simulink model "TV2016"  (Simulink 8.5)
settings: Solver=FixedStepDiscrete  StartTime=0.0  StopTime=inf  FixedStep=0.001  RelTol=1e-3
PreLoadFcn:
  | FSE_Parameters
values from neighbouring files (symbols this model uses):
  car_params = Simulink_Car_params    [TV2016_parameters.m]
  i_Diff = 15.47    [TV2016_parameters.m]
  Kp = 1    [TV2016_parameters.m]
  powerLimitControl = Simulink_el    [TV2016_parameters.m]
  settings = Simulink_Settings    [TV2016_parameters.m]
  SpdC_BCC = 0    [TV2016_parameters.m]
  Speed_Neg_sat = -21    [TV2016_parameters.m]
  Speed_Pos_sat = 21    [TV2016_parameters.m]
  speedEstimation = Simulink_speedEst    [TV2016_parameters.m]
  Tn_n = 0    [TV2016_parameters.m]
  tractionControl = Simulink_tc    [TV2016_parameters.m]
  Use_Joystick = 1    [TV2016_parameters.m]
  yawRateControl = Simulink_yawRate    [TV2016_parameters.m]
libraries: CarMaker4SL x174, simulink x27, simulink_extras x14
(part 2 of 5)

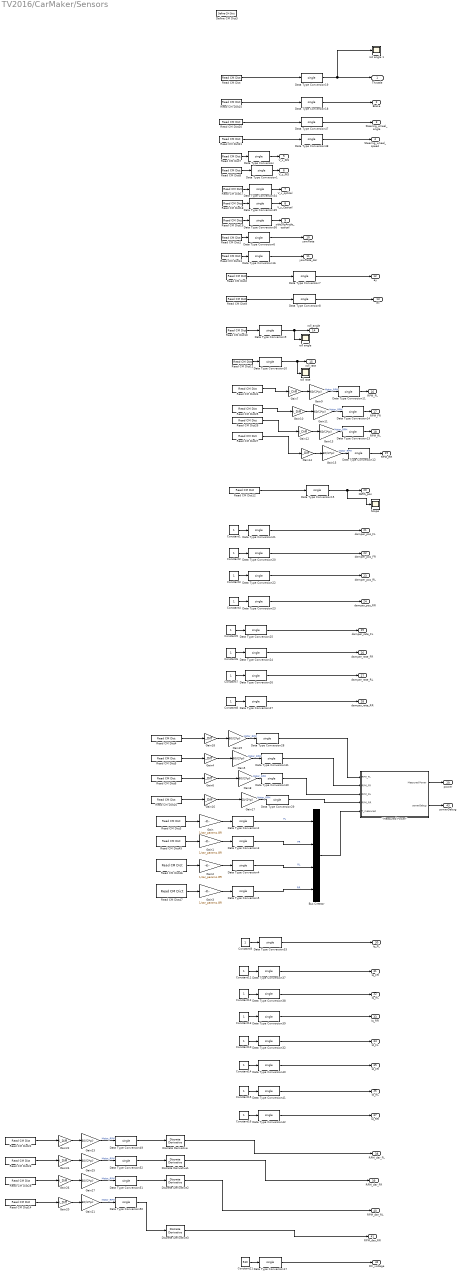
== system TV2016/CarMaker/Sensors  ==
  "\"Measured Power\"" : Subsystem
  Bus Creator : BusCreator  OutDataTypeStr=Bus: T_meas
      settings: InheritFromInputs=off
  Constant{1..16} (16 alike) : Constant
  Constant21 : Constant  Value=530
  Data Type Conversion{,1..42,47..52} (49 alike) : DataTypeConversion  OutDataTypeStr=single
  Define CM Dict3 : CarMaker4SL/Define CM Dict  xname=KERS_pos  xmono=off  xtype=Double  xdvaplace=None  xnstates=0  xfirststate=0  xinitial=0
  Discrete Derivative{,1..3} (4 alike) : simulink/Discrete/Discrete Derivative  gainval=1.0  ICPrevScaledInput=0.0  InputProcessing=Inherited  OutMin=[]  OutMax=[]  OutDataType=fixdt(1, 16)  OutScaling=2^-10  DoSatur=off
  Gain{,1..3} (4 alike) : Gain  Gain=1/car_params.GR
  Gain{4,6..7,10,12,14,16,18,20,22,24,26} (12 alike) : Gain  Gain=i_Diff
  Gain{5,8..9,11,13,15,17,19,21,23,25,27} (12 alike) : Gain  Gain=60/(2*pi)
  Read CM Dict : CarMaker4SL/Read CM Dict  xname=VC.Gas  xsync=off
  Read CM Dict1 : CarMaker4SL/Read CM Dict  xname=Vhcl.YawRate  xsync=off
  Read CM Dict10 : CarMaker4SL/Read CM Dict  xname=Vhcl.Roll  xsync=off
  Read CM Dict11 : CarMaker4SL/Read CM Dict  xname=Vhcl.RollVel  xsync=off
  Read CM Dict12 : CarMaker4SL/Read CM Dict  xname=KERS_pos  xsync=off
  Read CM Dict13 : CarMaker4SL/Read CM Dict  xname=Vhcl.YawAcc  xsync=off
  Read CM Dict14 : CarMaker4SL/Read CM Dict  xname=Car.WheelSpd_RR  xsync=off
  Read CM Dict15 : CarMaker4SL/Read CM Dict  xname=VC.Brake  xsync=off
  Read CM Dict16 : CarMaker4SL/Read CM Dict  xname=Car.WheelSpd_RR  xsync=off
  Read CM Dict17 : CarMaker4SL/Read CM Dict  xname=Car.vx  xsync=off
  Read CM Dict18 : CarMaker4SL/Read CM Dict  xname=Car.vy  xsync=off
  Read CM Dict19 : CarMaker4SL/Read CM Dict  xname=Car.SideSlipAngle  xsync=off
  Read CM Dict2 : CarMaker4SL/Read CM Dict  xname=Car.ay  xsync=off
  Read CM Dict20 : CarMaker4SL/Read CM Dict  xname=Vhcl.Steer.Ang  xsync=off
  Read CM Dict21 : CarMaker4SL/Read CM Dict  xname=Vhcl.Steer.Vel  xsync=off
  Read CM Dict22 : CarMaker4SL/Read CM Dict  xname=Car.WheelSpd_FL  xsync=off
  Read CM Dict23 : CarMaker4SL/Read CM Dict  xname=Car.WheelSpd_FR  xsync=off
  Read CM Dict24 : CarMaker4SL/Read CM Dict  xname=Car.WheelSpd_FL  xsync=off
  Read CM Dict25 : CarMaker4SL/Read CM Dict  xname=Car.WheelSpd_FR  xsync=off
  Read CM Dict26 : CarMaker4SL/Read CM Dict  xname=Car.WheelSpd_RL  xsync=off
  Read CM Dict27 : CarMaker4SL/Read CM Dict  xname=Car.WheelSpd_RR  xsync=off
  Read CM Dict28 : CarMaker4SL/Read CM Dict  xname=Car.WheelSpd_RL  xsync=off
  Read CM Dict3 : CarMaker4SL/Read CM Dict  xname=PT.WFL.Trq_Drive  xsync=off
  Read CM Dict4 : CarMaker4SL/Read CM Dict  xname=Car.WheelSpd_FL  xsync=off
  Read CM Dict45 : CarMaker4SL/Read CM Dict  xname=PT.WFR.Trq_Drive  xsync=off
  Read CM Dict46 : CarMaker4SL/Read CM Dict  xname=PT.WRL.Trq_Drive  xsync=off
  Read CM Dict47 : CarMaker4SL/Read CM Dict  xname=PT.WRR.Trq_Drive  xsync=off
  Read CM Dict5 : CarMaker4SL/Read CM Dict  xname=Car.WheelSpd_FR  xsync=off
  Read CM Dict6 : CarMaker4SL/Read CM Dict  xname=Car.WheelSpd_RL  xsync=off
  Read CM Dict7 : CarMaker4SL/Read CM Dict  xname=Car.vx  xsync=off
  Read CM Dict8 : CarMaker4SL/Read CM Dict  xname=Car.vy  xsync=off
  Read CM Dict9 : CarMaker4SL/Read CM Dict  xname=Car.ax  xsync=off
  Scope : Scope
      settings: SaveName=ScopeData77
  "roll angle " : Scope
      settings: ShowLegends=on  YMin=-17.5  YMax=17.5  SaveName=ScopeData63
  roll angle 1 : Scope
      settings: ShowLegends=on  YMin=-17.5  YMax=17.5  SaveName=ScopeData78
  roll rate : Scope
      settings: ShowLegends=on  YMin=-17.5  YMax=17.5  SaveName=ScopeData65
  "Throttle " : Outport
  "Brake " : Outport  Port=2
  "Steering_wheel_angle " : Outport  Port=3
  Steering_wheel_speed : Outport  Port=4
  V_x_INS : Outport  Port=5
  V_y_INS : Outport  Port=6
  V_x_optical : Outport  Port=7
  V_y_Optical : Outport  Port=8
  sideSlipAngle_optical : Outport  Port=9
  yawRate : Outport  Port=10
  yawRate_der : Outport  Port=11
  ay : Outport  Port=12
  "ax " : Outport  Port=13
  roll_angle : Outport  Port=14
  roll_rate : Outport  Port=15
  RPM_FL : Outport  Port=16
  RPM_FR : Outport  Port=17
  RPM_RL : Outport  Port=18
  RPM_RR : Outport  Port=19
  KERS_pos : Outport  Port=20
  damper_pos_FL : Outport  Port=21
  damper_pos_FR : Outport  Port=22
  damper_pos_RL : Outport  Port=23
  damper_pos_RR : Outport  Port=24
  damper_rate_FL : Outport  Port=25
  damper_rate_FR : Outport  Port=26
  damper_rate_RL : Outport  Port=27
  damper_rate_RR : Outport  Port=28
  power : Outport  Port=29
  Iq_FL : Outport  Port=30
  Iq_FR : Outport  Port=31
  Iq_RL : Outport  Port=32
  Iq_RR : Outport  Port=33
  Id_FL : Outport  Port=34
  Id_FR : Outport  Port=35
  Id_RL : Outport  Port=36
  Id_RR : Outport  Port=37
  RPM_der_FL : Outport  Port=38
  RPM_der_FR : Outport  Port=39
  RPM_der_RL : Outport  Port=40
  RPM_der_RR : Outport  Port=41
  DC_voltage : Outport  Port=42
  powerDebug : Outport  Port=43
  wires:
  Read CM Dict7/1 -> Data Type Conversion/1
  Read CM Dict8/1 -> Data Type Conversion1/1
  Read CM Dict1/1 -> Data Type Conversion6/1
  Data Type Conversion/1 -> V_x_INS/1
  Data Type Conversion1/1 -> V_y_INS/1
  Data Type Conversion6/1 -> yawRate/1
  Read CM Dict10/1 -> Data Type Conversion9/1
  Data Type Conversion9/1 -> "roll angle "/1, roll_angle/1
  Read CM Dict11/1 -> Data Type Conversion10/1
  Data Type Conversion10/1 -> roll rate/1, roll_rate/1
  Gain7/1 -> Gain9/1
  Read CM Dict24/1 -> Gain7/1
  Read CM Dict25/1 -> Gain10/1
  Gain10/1 -> Gain11/1
  Gain12/1 -> Gain13/1
  Gain14/1 -> Gain15/1
  Read CM Dict26/1 -> Gain12/1
  Read CM Dict27/1 -> Gain14/1
  Gain9/1 -> Data Type Conversion11/1  "Motor_RPM"
  Gain15/1 -> Data Type Conversion12/1  "Motor_RPM"
  Gain13/1 -> Data Type Conversion13/1  "Motor_RPM"
  Gain11/1 -> Data Type Conversion14/1  "Motor_RPM"
  Data Type Conversion11/1 -> RPM_FL/1
  Data Type Conversion14/1 -> RPM_FR/1
  Data Type Conversion13/1 -> RPM_RL/1
  Data Type Conversion12/1 -> RPM_RR/1
  Read CM Dict12/1 -> Data Type Conversion15/1
  Data Type Conversion15/1 -> Scope/1, KERS_pos/1
  Data Type Conversion7/1 -> ay/1
  Data Type Conversion8/1 -> "ax "/1
  Read CM Dict/1 -> Data Type Conversion19/1
  Read CM Dict15/1 -> Data Type Conversion18/1
  Data Type Conversion18/1 -> "Brake "/1
  Data Type Conversion19/1 -> roll angle 1/1, "Throttle "/1
  Data Type Conversion21/1 -> damper_pos_FL/1
  Constant1/1 -> Data Type Conversion21/1
  Data Type Conversion20/1 -> damper_pos_FR/1
  Constant2/1 -> Data Type Conversion20/1
  Data Type Conversion22/1 -> damper_pos_RL/1
  Constant3/1 -> Data Type Conversion22/1
  Data Type Conversion23/1 -> damper_pos_RR/1
  Constant4/1 -> Data Type Conversion23/1
  Data Type Conversion25/1 -> damper_rate_FL/1
  Constant5/1 -> Data Type Conversion25/1
  Data Type Conversion24/1 -> damper_rate_FR/1
  Constant6/1 -> Data Type Conversion24/1
  Data Type Conversion26/1 -> damper_rate_RL/1
  Constant7/1 -> Data Type Conversion26/1
  Data Type Conversion27/1 -> damper_rate_RR/1
  Constant8/1 -> Data Type Conversion27/1
  Read CM Dict3/1 -> Gain/1
  Read CM Dict45/1 -> Gain1/1
  Read CM Dict46/1 -> Gain2/1
  Read CM Dict47/1 -> Gain3/1
  Data Type Conversion2/1 -> Bus Creator/1  "FL"
  Data Type Conversion3/1 -> Bus Creator/2  "FR"
  Data Type Conversion4/1 -> Bus Creator/3  "RL"
  Data Type Conversion5/1 -> Bus Creator/4  "RR"
  Gain/1 -> Data Type Conversion2/1
  Gain1/1 -> Data Type Conversion3/1
  Gain2/1 -> Data Type Conversion4/1
  Gain3/1 -> Data Type Conversion5/1
  Bus Creator/1 -> "\"Measured Power\""/5(T_measured)
  Gain18/1 -> Gain19/1
  Read CM Dict4/1 -> Gain18/1
  Read CM Dict5/1 -> Gain4/1
  Gain4/1 -> Gain5/1
  Gain6/1 -> Gain8/1
  Gain16/1 -> Gain17/1
  Read CM Dict6/1 -> Gain6/1
  Read CM Dict16/1 -> Gain16/1
  Gain19/1 -> Data Type Conversion28/1  "Motor_RPM"
  Gain17/1 -> Data Type Conversion29/1  "Motor_RPM"
  Gain8/1 -> Data Type Conversion30/1  "Motor_RPM"
  Gain5/1 -> Data Type Conversion31/1  "Motor_RPM"
  Data Type Conversion29/1 -> "\"Measured Power\""/4(RPM_RR)
  Data Type Conversion30/1 -> "\"Measured Power\""/3(RPM_RL)
  Data Type Conversion31/1 -> "\"Measured Power\""/2(RPM_FR)
  Data Type Conversion28/1 -> "\"Measured Power\""/1(RPM_FL)
  "\"Measured Power\""/1("Measured Power ") -> power/1
  "\"Measured Power\""/2(powerDebug) -> powerDebug/1
  Data Type Conversion33/1 -> Iq_FL/1
  Constant9/1 -> Data Type Conversion33/1
  Data Type Conversion32/1 -> Id_FL/1
  Constant10/1 -> Data Type Conversion32/1
  Read CM Dict9/1 -> Data Type Conversion8/1
  Read CM Dict2/1 -> Data Type Conversion7/1
  Read CM Dict17/1 -> Data Type Conversion34/1
  Read CM Dict18/1 -> Data Type Conversion35/1
  Data Type Conversion34/1 -> V_x_optical/1
  Data Type Conversion35/1 -> V_y_Optical/1
  Data Type Conversion36/1 -> sideSlipAngle_optical/1
  Read CM Dict19/1 -> Data Type Conversion36/1
  Data Type Conversion37/1 -> Iq_FR/1
  Constant11/1 -> Data Type Conversion37/1
  Data Type Conversion38/1 -> Iq_RL/1
  Constant12/1 -> Data Type Conversion38/1
  Data Type Conversion39/1 -> Iq_RR/1
  Constant13/1 -> Data Type Conversion39/1
  Data Type Conversion40/1 -> Id_FR/1
  Constant14/1 -> Data Type Conversion40/1
  Data Type Conversion41/1 -> Id_RL/1
  Constant15/1 -> Data Type Conversion41/1
  Data Type Conversion42/1 -> Id_RR/1
  Constant16/1 -> Data Type Conversion42/1
  Read CM Dict20/1 -> Data Type Conversion47/1
  Read CM Dict21/1 -> Data Type Conversion48/1
  Data Type Conversion47/1 -> "Steering_wheel_angle "/1
  Data Type Conversion48/1 -> Steering_wheel_speed/1
  Data Type Conversion16/1 -> yawRate_der/1
  Read CM Dict13/1 -> Data Type Conversion16/1
  Data Type Conversion17/1 -> DC_voltage/1
  Constant21/1 -> Data Type Conversion17/1
  Gain22/1 -> Gain23/1
  Read CM Dict22/1 -> Gain22/1
  Read CM Dict23/1 -> Gain24/1
  Gain24/1 -> Gain25/1
  Gain26/1 -> Gain27/1
  Gain20/1 -> Gain21/1
  Read CM Dict28/1 -> Gain26/1
  Read CM Dict14/1 -> Gain20/1
  Gain23/1 -> Data Type Conversion49/1  "Motor_RPM"
  Gain21/1 -> Data Type Conversion50/1  "Motor_RPM"
  Gain27/1 -> Data Type Conversion51/1  "Motor_RPM"
  Gain25/1 -> Data Type Conversion52/1  "Motor_RPM"
  Data Type Conversion50/1 -> Discrete Derivative3/1
  Data Type Conversion51/1 -> Discrete Derivative2/1
  Data Type Conversion52/1 -> Discrete Derivative1/1
  Data Type Conversion49/1 -> Discrete Derivative/1
  Discrete Derivative/1 -> RPM_der_FL/1
  Discrete Derivative1/1 -> RPM_der_FR/1
  Discrete Derivative2/1 -> RPM_der_RL/1
  Discrete Derivative3/1 -> RPM_der_RR/1

== system TV2016/CarMaker/VehicleControl ==
  note: <Your model here>
  note: When implementing a vehicle control model,
      | be sure to add '-disablevehiclecontrol' to the command line arguments
      | in the CarMaker Model Configuration block.
      | Otherwise your model will possibly not see the original DrivMan signals
      | on its inputs, but those of a currently activated C-coded vehicle control model instead.
  Sync_In : Inport
  DrivMan.In : Inport  Port=2
  Bus Creator2 : BusCreator  Inputs=2
  CreateBus Vhcl.Misc : Subsystem
  CreateBus Vhcl.Wheel.In : Subsystem
  CreateBus VhclCtrl : Subsystem
  CreateBus VhclCtrl.PT : Subsystem
  CreateBus VhclCtrl.Steering : Subsystem
  Demux2 : Demux  Outputs=2
  VehicleControl : S-Function  FunctionName=CM_Sfun  Parameters='VehicleControl'
  VehicleControlUpd : S-Function  FunctionName=CM_Sfun  Parameters='VehicleControlUpd'
  Sync_Out : Outport
  Vhcl.Model.Source : Outport  Port=2
  VhclCtrl.Steering : Outport  Port=3
  Vhcl.Wheel.In : Outport  Port=4
  Vhcl.Misc : Outport  Port=5
  VhclCtrl.Brake : Outport  Port=6
  VhclCtrl.PT : Outport  Port=7
  wires:
  CreateBus VhclCtrl/1(Out) -> VehicleControlUpd/2
  VehicleControl/2 -> CreateBus VhclCtrl/1(In)
  VehicleControlUpd/2 -> Vhcl.Model.Source/1
  VehicleControlUpd/4 -> CreateBus Vhcl.Wheel.In/1(In1)
  VehicleControlUpd/5 -> CreateBus Vhcl.Misc/1(In1)
  VehicleControlUpd/6 -> Demux2/1
  VehicleControlUpd/7 -> CreateBus VhclCtrl.PT/1(In1)
  VehicleControlUpd/3 -> CreateBus VhclCtrl.Steering/1(In1)
  CreateBus Vhcl.Misc/1(Out1) -> Vhcl.Misc/1
  CreateBus Vhcl.Wheel.In/1(Out1) -> Vhcl.Wheel.In/1
  DrivMan.In/1 -> VehicleControl/2
  VehicleControl/1 -> VehicleControlUpd/1
  Sync_In/1 -> VehicleControl/1
  CreateBus VhclCtrl.PT/1(Out1) -> VhclCtrl.PT/1
  Bus Creator2/1 -> VhclCtrl.Brake/1
  CreateBus VhclCtrl.Steering/1(Out1) -> VhclCtrl.Steering/1
  VehicleControlUpd/1 -> Sync_Out/1
  Demux2/2 -> Bus Creator2/2  "VhclCtrl BrakePark"
  Demux2/1 -> Bus Creator2/1  "VhclCtrl Brake"

== system TV2016/CarMaker/Control_System /Control  ==
  "States " : Inport
  Bus Creator : BusCreator  OutDataTypeStr=Bus: Ti_lim  NonVirtualBus=on
      settings: InheritFromInputs=off
  Bus Selector : BusSelector  OutputSignals=FL,FR,RL,RR
  "Power Limit Torque Reduction Controller " : Subsystem
  Product{1..3,5} (4 alike) : Product
  Red factor : Scope
      settings: ShowLegends=on  TimeRange=10  YMin=0.625  YMax=1  SaveName=ScopeData26
  Red factor1 : Scope
      settings: ShowLegends=on  TimeRange=10  YMin=21  YMax=21  SaveName=ScopeData45
  Red factor2 : Scope
      settings: ShowLegends=on  TimeRange=10  YMin=19.95  YMax=22.05  SaveName=ScopeData58
  "Slip Rate Control " : Subsystem
  Throttle / Brake Mapping : Subsystem
  "Torque allocation " : Subsystem
  "Yaw Rate Controller " : Subsystem
  Ti_lim : Outport
  Mz_ref : Outport  Port=2
  T_req : Outport  Port=3
  r_ref : Outport  Port=4
  Mz_error : Outport  Port=5
  wires:
  "Yaw Rate Controller "/4(Mz_ref) -> Mz_ref/1, "Torque allocation "/1(Mz_ref)
  "States "/1 -> "Yaw Rate Controller "/1(States), "Slip Rate Control "/2("States "), "Power Limit Torque Reduction Controller "/1(states), "Torque allocation "/3("States "), Throttle / Brake Mapping/1("states ")
  "Torque allocation "/1(Ti_lim) -> "Slip Rate Control "/1(Ti_ref)
  Throttle / Brake Mapping/1(T_req) -> "Slip Rate Control "/3(T_req), "Torque allocation "/2(T_req), T_req/1
  "Yaw Rate Controller "/1("r_ref ") -> r_ref/1  "r_ref"
  "Slip Rate Control "/1(Ti_lim) -> Bus Selector/1
  Bus Selector/4 -> Product3/2, Red factor1/1  "<RR>"
  Bus Selector/3 -> Product1/2  "<RL>"
  Bus Selector/2 -> Product2/2  "<FR>"
  Bus Selector/1 -> Product5/2  "<FL>"
  Product5/1 -> Bus Creator/1  "FL"
  Product2/1 -> Bus Creator/2  "FR"
  Product1/1 -> Bus Creator/3  "RL"
  Product3/1 -> Red factor2/1, Bus Creator/4  "RR"
  "Power Limit Torque Reduction Controller "/1(Reduction Factor) -> Product2/1, Product5/1, Product1/1, Product3/1, Red factor/1
  Bus Creator/1 -> Ti_lim/1
  "Torque allocation "/2("Mz_error ") -> "Yaw Rate Controller "/2("Mz_error "), Mz_error/1

== system TV2016/CarMaker/Control_System /Output Interface  ==
  states : Inport
  Ti_lim : Inport  Port=2
  MATLAB Function : MATLAB Function  TreatAsAtomicUnit=on
  "Ti_pos " : Outport
  Ti_neg : Outport  Port=2
  wi_setpoints : Outport  Port=3
  wires:
  MATLAB Function/2(Ti_neg) -> Ti_neg/1
  Ti_lim/1 -> MATLAB Function/1(Ti)
  MATLAB Function/1(Ti_pos) -> "Ti_pos "/1
  MATLAB Function/3(wi_setpoints) -> wi_setpoints/1
  states/1 -> MATLAB Function/2(states)

== system TV2016/CarMaker/Debug Information /Motor Rpm log   ==
  Abs : Abs
  Discrete Derivative : simulink/Discrete/Discrete Derivative  gainval=1.0  ICPrevScaledInput=0.0  InputProcessing=Inherited  OutMin=[]  OutMax=[]  OutDataType=fixdt(1, 16)  OutScaling=2^-10  DoSatur=off
  Fl_derivate : Scope
      settings: ShowLegends=on  TimeRange=3.722  YMin=0  YMax=10000  SaveName=ScopeData57
  Gain{7,10,12,14} (4 alike) : Gain  Gain=i_Diff
  Gain{9,11,13,15} (4 alike) : Gain  Gain=60/(2*pi)
  Mux1 : Mux
  Rate Transition : RateTransition  OutPortSampleTime=settings.control_system_sample_time
  Read CM Dict24 : CarMaker4SL/Read CM Dict  xname=Car.WheelSpd_FL  xsync=off
  Read CM Dict25 : CarMaker4SL/Read CM Dict  xname=Car.WheelSpd_FR  xsync=off
  Read CM Dict26 : CarMaker4SL/Read CM Dict  xname=Car.WheelSpd_RL  xsync=off
  Read CM Dict27 : CarMaker4SL/Read CM Dict  xname=Car.WheelSpd_RR  xsync=off
  Saturation : Saturate  UpperLimit=50000
  To File : ToFile  Filename=MAT_files\MotorRPMS.mat  MatrixName=MotorRpms  SaveFormat=Timeseries
  eng rot : Scope
      settings: ShowLegends=on  TimeRange=0.03226232678936204  YMin=358.5090361445784  YMax=366.6415662650603  SaveName=ScopeData55
  wires:
  Gain7/1 -> Gain9/1
  Gain9/1 -> Mux1/1, Rate Transition/1  "Motor_RPM"
  Read CM Dict24/1 -> Gain7/1
  Read CM Dict25/1 -> Gain10/1
  Gain10/1 -> Gain11/1
  Gain11/1 -> Mux1/2  "Motor_RPM"
  Gain12/1 -> Gain13/1
  Gain13/1 -> Mux1/3  "Motor_RPM"
  Gain14/1 -> Gain15/1
  Gain15/1 -> Mux1/4  "Motor_RPM"
  Read CM Dict26/1 -> Gain12/1
  Read CM Dict27/1 -> Gain14/1
  Mux1/1 -> eng rot/1, To File/1
  Discrete Derivative/1 -> Abs/1
  Abs/1 -> Saturation/1
  Saturation/1 -> Fl_derivate/1
  Rate Transition/1 -> Discrete Derivative/1

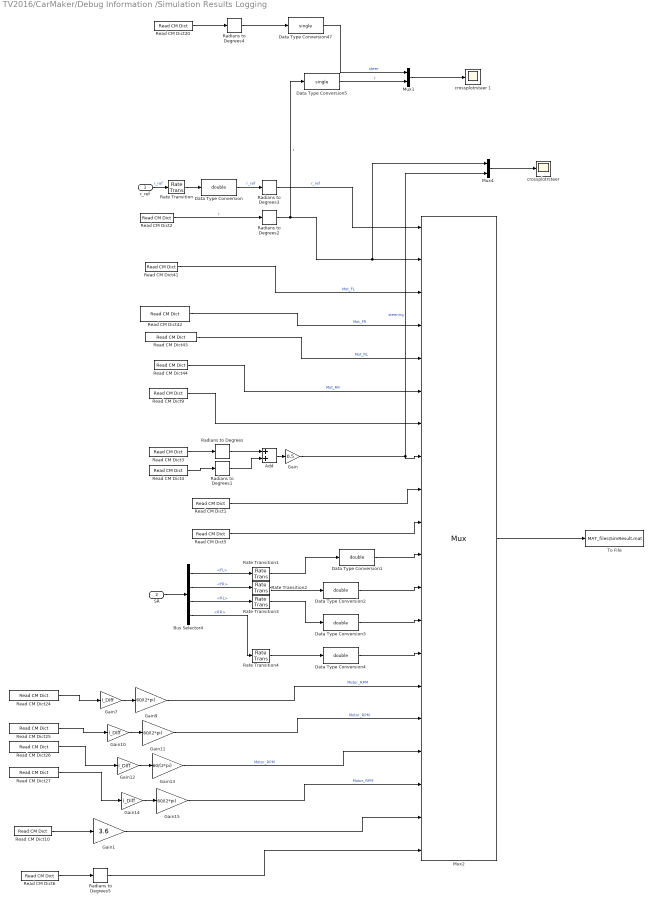
== system TV2016/CarMaker/Debug Information /Simulation Results Logging ==
  r_ref : Inport
  SR : Inport  Port=2
  Add : Sum
  Bus Selector4 : BusSelector  OutputSignals=FL,FR,RL,RR
  Data Type Conversion{,1..4} (5 alike) : DataTypeConversion  OutDataTypeStr=double
  Data Type Conversion47 : DataTypeConversion  OutDataTypeStr=single
  Data Type Conversion5 : DataTypeConversion  OutDataTypeStr=single
  Gain : Gain  Gain=0.5
  Gain1 : Gain  Gain=3.6
  Gain{7,10,12,14} (4 alike) : Gain  Gain=i_Diff
  Gain{9,11,13,15} (4 alike) : Gain  Gain=60/(2*pi)
  Mux1 : Mux  Inputs=2
  Mux2 : Mux  Inputs=20
  Mux4 : Mux  Inputs=2
  Radians to Degrees{,1..5} (6 alike) : simulink_extras/Transformations/Radians to Degrees
  Rate Transition{,1..4} (5 alike) : RateTransition  OutPortSampleTime=0.001
  Read CM Dict1 : CarMaker4SL/Read CM Dict  xname=Vhcl.Fr1.x  xsync=off
  Read CM Dict10 : CarMaker4SL/Read CM Dict  xname=Car.vx  xsync=off
  Read CM Dict2 : CarMaker4SL/Read CM Dict  xname=Car.YawRate  xsync=off
  Read CM Dict20 : CarMaker4SL/Read CM Dict  xname=Vhcl.Steer.Ang  xsync=off
  Read CM Dict24 : CarMaker4SL/Read CM Dict  xname=Car.WheelSpd_FL  xsync=off
  Read CM Dict25 : CarMaker4SL/Read CM Dict  xname=Car.WheelSpd_FR  xsync=off
  Read CM Dict26 : CarMaker4SL/Read CM Dict  xname=Car.WheelSpd_RL  xsync=off
  Read CM Dict27 : CarMaker4SL/Read CM Dict  xname=Car.WheelSpd_RR  xsync=off
  Read CM Dict3 : CarMaker4SL/Read CM Dict  xname=Car.CFR.rz  xsync=off
  Read CM Dict4 : CarMaker4SL/Read CM Dict  xname=Car.CFL.rz  xsync=off
  Read CM Dict41 : CarMaker4SL/Read CM Dict  xname=PT.WFL.Trq_Drive  xsync=off
  Read CM Dict42 : CarMaker4SL/Read CM Dict  xname=PT.WFR.Trq_Drive  xsync=off
  Read CM Dict43 : CarMaker4SL/Read CM Dict  xname=PT.WRL.Trq_Drive  xsync=off
  Read CM Dict44 : CarMaker4SL/Read CM Dict  xname=PT.WRR.Trq_Drive  xsync=off
  Read CM Dict5 : CarMaker4SL/Read CM Dict  xname=Vhcl.Fr1.y  xsync=off
  Read CM Dict6 : CarMaker4SL/Read CM Dict  xname=Vhcl.Steer.Ang  xsync=off
  Read CM Dict9 : CarMaker4SL/Read CM Dict  xname=Car.ay  xsync=off
  To File : ToFile  Filename=MAT_files\SimResult.mat  MatrixName=sim  SaveFormat=Timeseries
  "crossplotrsteer " : Scope
      settings: ShowLegends=on  TimeRange=0.01155166537365709  YMin=3.631313131313132  YMax=5.196969696969697  SaveName=ScopeData76
  crossplotrsteer 1 : Scope
      settings: ShowLegends=on  TimeRange=0.6169191083805927  YMin=-0.9397630019749759  YMax=0.9205440761112005  SaveName=ScopeData32
  wires:
  r_ref/1 -> Rate Transition/1  "r_ref"
  Read CM Dict2/1 -> Radians to Degrees2/1  "r"
  Data Type Conversion/1 -> Radians to Degrees3/1  "r_ref"
  Read CM Dict42/1 -> Mux2/4  "Mot_FR"
  Read CM Dict43/1 -> Mux2/5  "Mot_RL"
  Read CM Dict41/1 -> Mux2/3  "Mot_FL"
  Read CM Dict44/1 -> Mux2/6  "Mot_RR"
  Read CM Dict9/1 -> Mux2/7
  Read CM Dict3/1 -> Radians to Degrees/1
  Read CM Dict4/1 -> Radians to Degrees1/1
  Radians to Degrees/1 -> Add/1
  Radians to Degrees1/1 -> Add/2
  Radians to Degrees2/1 -> Mux4/1, Mux2/2, Data Type Conversion5/1  "r"
  Radians to Degrees3/1 -> Mux2/1  "r_ref"
  Add/1 -> Gain/1
  Mux2/1 -> To File/1
  Read CM Dict1/1 -> Mux2/9
  Read CM Dict5/1 -> Mux2/10
  Rate Transition/1 -> Data Type Conversion/1
  Mux4/1 -> "crossplotrsteer "/1
  Gain/1 -> Mux2/8, Mux4/2  "steering"
  Bus Selector4/1 -> Rate Transition1/1  "<FL>"
  Bus Selector4/2 -> Rate Transition2/1  "<FR>"
  Bus Selector4/3 -> Rate Transition3/1  "<RL>"
  Bus Selector4/4 -> Rate Transition4/1  "<RR>"
  SR/1 -> Bus Selector4/1
  Rate Transition1/1 -> Data Type Conversion1/1
  Rate Transition2/1 -> Data Type Conversion2/1
  Rate Transition3/1 -> Data Type Conversion3/1
  Rate Transition4/1 -> Data Type Conversion4/1
  Data Type Conversion1/1 -> Mux2/11
  Data Type Conversion2/1 -> Mux2/12
  Data Type Conversion3/1 -> Mux2/13
  Data Type Conversion4/1 -> Mux2/14
  Gain7/1 -> Gain9/1
  Gain9/1 -> Mux2/15  "Motor_RPM"
  Read CM Dict24/1 -> Gain7/1
  Read CM Dict25/1 -> Gain10/1
  Gain10/1 -> Gain11/1
  Gain11/1 -> Mux2/16  "Motor_RPM"
  Gain12/1 -> Gain13/1
  Gain13/1 -> Mux2/17  "Motor_RPM"
  Gain14/1 -> Gain15/1
  Gain15/1 -> Mux2/18  "Motor_RPM"
  Read CM Dict26/1 -> Gain12/1
  Read CM Dict27/1 -> Gain14/1
  Read CM Dict10/1 -> Gain1/1
  Gain1/1 -> Mux2/19
  Read CM Dict20/1 -> Radians to Degrees4/1
  Data Type Conversion47/1 -> Mux1/1  "steer"
  Mux1/1 -> crossplotrsteer 1/1
  Radians to Degrees4/1 -> Data Type Conversion47/1
  Data Type Conversion5/1 -> Mux1/2  "r"
  Read CM Dict6/1 -> Radians to Degrees5/1
  Radians to Degrees5/1 -> Mux2/20

== system TV2016/CarMaker/Estimations/EstimateVx ==
  sensors : Inport
  Fz_est : Inport  Port=2
  velocity_Estimation : MATLAB Function  TreatAsAtomicUnit=on
  v_x_est : Outport
  wires:
  sensors/1 -> velocity_Estimation/1(sensors)
  Fz_est/1 -> velocity_Estimation/2(normalForces)
  velocity_Estimation/1(V_est_x) -> v_x_est/1

== system TV2016/CarMaker/Estimations/Fx_Estimation ==
  sensors : Inport
  T_CM : Inport  Port=2
  EstimateFx : MATLAB Function  TreatAsAtomicUnit=on
  Fx : Outport
  wires:
  sensors/1 -> EstimateFx/1(sensors)
  EstimateFx/1(Fx) -> Fx/1
  T_CM/1 -> EstimateFx/2(T_CM)

== system TV2016/CarMaker/Estimations/Fz_Estimation ==
  sensors : Inport
  v_x : Inport  Port=2
  Bus Selector : BusSelector  OutputSignals=damper_rate_FL,damper_rate_FR,damper_rate_RL,damper_rate_RR
  Constant : Constant  Value=settings.select_Fz_est_method
  DamperRateLookup{,1..3} (4 alike) : Lookup_n-D  NumberOfTableDimensions=1  BreakpointsForDimension1=single([-250,0,250]);  Table=single([-900,0,900]);  InternalRulePriority=Speed  RndMeth=Simplest  InputSameDT=on
  FzEstDamper : MATLAB Function  TreatAsAtomicUnit=on
  FzEstLoadTransfer : MATLAB Function  TreatAsAtomicUnit=on
  Index Vector : MultiPortSwitch  Inputs=2
  Fz_est : Outport
  Fz_LoadTransfer_est : Outport  Port=2
  Fz_damper_est : Outport  Port=3
  wires:
  sensors/1 -> FzEstDamper/1(sensors), Bus Selector/1, FzEstLoadTransfer/1(sensor)
  FzEstLoadTransfer/1(Fz_loadTransfer_est) -> Fz_LoadTransfer_est/1, Index Vector/2
  DamperRateLookup/1 -> FzEstDamper/2(Fz_damp_FL)  "Fz_damp_FL"
  Bus Selector/1 -> DamperRateLookup/1  "<damper_rate_FL>"
  Bus Selector/2 -> DamperRateLookup1/1  "<damper_rate_FR>"
  Bus Selector/3 -> DamperRateLookup2/1  "<damper_rate_RL>"
  Bus Selector/4 -> DamperRateLookup3/1  "<damper_rate_RR>"
  DamperRateLookup1/1 -> FzEstDamper/3(Fz_damp_FR)
  DamperRateLookup2/1 -> FzEstDamper/4(Fz_damp_RL)
  DamperRateLookup3/1 -> FzEstDamper/5(Fz_damp_RR)
  FzEstDamper/1(Fz_damper_est) -> Index Vector/3, Fz_damper_est/1
  Constant/1 -> Index Vector/1
  Index Vector/1 -> Fz_est/1
  v_x/1 -> FzEstLoadTransfer/2(vx)

== system TV2016/CarMaker/Estimations/RPM_to_linearVelocity ==
  sensors : Inport
  meanWheelAngle : Inport  Port=2
  whl_v_calculation : MATLAB Function  TreatAsAtomicUnit=on
  whl_speed : Outport
  wires:
  whl_v_calculation/1(whl_speed) -> whl_speed/1
  sensors/1 -> whl_v_calculation/1(sensors)
  meanWheelAngle/1 -> whl_v_calculation/2(meanWheelAngle)

== system TV2016/CarMaker/Estimations/SR_Calculation ==
  v_x : Inport
  whl_v : Inport  Port=2
  sensorInput : Inport  Port=3
  Slip ratio : MATLAB Function  TreatAsAtomicUnit=on
  SR : Outport
  wires:
  v_x/1 -> Slip ratio/1(V_x)
  Slip ratio/1(SR) -> SR/1
  whl_v/1 -> Slip ratio/2(whl_v)
  sensorInput/1 -> Slip ratio/3(sensor)

== system TV2016/CarMaker/Estimations/calculateMeanWheelAngle ==
  sensorInput : Inport
  calculateWheelangleandSpeed : MATLAB Function  TreatAsAtomicUnit=on
  mean_wheel_angle : Outport
  mean_wheel_speed : Outport  Port=2
  wires:
  sensorInput/1 -> calculateWheelangleandSpeed/1(sensor)
  calculateWheelangleandSpeed/1(mean_wheel_angle) -> mean_wheel_angle/1
  calculateWheelangleandSpeed/2(mean_wheel_speed) -> mean_wheel_speed/1

== system TV2016/CarMaker/Estimations/createStateBus ==
  mean_wheel_angle : Inport
  mean_wheel_speed : Inport  Port=2
  Fz_CM : Inport  Port=3
  Fx : Inport  Port=4
  sensors : Inport  Port=5
  Fz_est : Inport  Port=6
  whl_speed_cog : Inport  Port=7
  v_x : Inport  Port=8
  v_y : Inport  Port=9
  SR : Inport  Port=10
  frictionCoefficient : Inport  Port=11
  Bus Creator1 : BusCreator  Inputs=35  OutDataTypeStr=Bus: States  NonVirtualBus=on
      settings: InheritFromInputs=off
  Bus Selector{,2..4} (4 alike) : BusSelector  OutputSignals=FL,FR,RL,RR
  Bus Selector1 : BusSelector  OutputSignals=Input_throttle,Input_brake,KERS_pos,sideSlipAngle_optical,yawRate,yawRate_der,ax,ay,RPM_FL,RPM_FR,RPM_RL,RPM_RR,power,DC_voltage
  Constant : Constant  Value=settings.use_estimated_Fz
  Index Vector : MultiPortSwitch  DataPortOrder=Zero-based contiguous  Inputs=2  zeroidx=on
  states : Outport
  wires:
  sensors/1 -> Bus Selector1/1
  Fz_est/1 -> Index Vector/3
  Fz_CM/1 -> Index Vector/2
  Constant/1 -> Index Vector/1
  Index Vector/1 -> Bus Selector/1
  whl_speed_cog/1 -> Bus Selector2/1
  Fx/1 -> Bus Selector3/1
  SR/1 -> Bus Selector4/1
  Bus Creator1/1 -> states/1
  Bus Selector1/10 -> Bus Creator1/10  "<RPM_FR>"
  Bus Selector1/9 -> Bus Creator1/9  "<RPM_FL>"
  Bus Selector1/11 -> Bus Creator1/11  "<RPM_RL>"
  Bus Selector1/8 -> Bus Creator1/8  "<ay>"
  Bus Selector1/12 -> Bus Creator1/12  "<RPM_RR>"
  Bus Selector1/7 -> Bus Creator1/7  "<ax>"
  Bus Selector1/13 -> Bus Creator1/13  "<power>"
  Bus Selector1/6 -> Bus Creator1/6  "<yawRate_der>"
  Bus Selector1/14 -> Bus Creator1/14  "<DC_voltage>"
  Bus Selector1/5 -> Bus Creator1/5  "<yawRate>"
  Bus Selector1/4 -> Bus Creator1/4  "<sideSlipAngle_optical>"
  Bus Selector1/3 -> Bus Creator1/3  "<KERS_pos>"
  Bus Selector1/2 -> Bus Creator1/2  "<Input_brake>"
  Bus Selector1/1 -> Bus Creator1/1  "<Input_throttle>"
  mean_wheel_angle/1 -> Bus Creator1/15
  mean_wheel_speed/1 -> Bus Creator1/16
  v_x/1 -> Bus Creator1/17
  v_y/1 -> Bus Creator1/18
  Bus Selector/1 -> Bus Creator1/23  "<FL>"
  Bus Selector/2 -> Bus Creator1/24  "<FR>"
  Bus Selector/3 -> Bus Creator1/25  "<RL>"
  Bus Selector/4 -> Bus Creator1/26  "<RR>"
  Bus Selector2/1 -> Bus Creator1/27  "<FL>"
  Bus Selector2/2 -> Bus Creator1/28  "<FR>"
  Bus Selector2/3 -> Bus Creator1/29  "<RL>"
  Bus Selector2/4 -> Bus Creator1/30  "<RR>"
  Bus Selector4/1 -> Bus Creator1/31  "<FL>"
  Bus Selector4/2 -> Bus Creator1/32  "<FR>"
  Bus Selector4/3 -> Bus Creator1/33  "<RL>"
  Bus Selector4/4 -> Bus Creator1/34  "<RR>"
  Bus Selector3/1 -> Bus Creator1/19  "<FL>"
  Bus Selector3/2 -> Bus Creator1/20  "<FR>"
  Bus Selector3/3 -> Bus Creator1/21  "<RL>"
  Bus Selector3/4 -> Bus Creator1/22  "<RR>"
  frictionCoefficient/1 -> Bus Creator1/35

== system TV2016/CarMaker/Estimations/friction_estimation ==
  Fx : Inport
  SR : Inport  Port=2
  Fz : Inport  Port=3
  estimateFrictionCoefficient : MATLAB Function  TreatAsAtomicUnit=on
  mu : Outport
  normLongTireForce : Outport  Port=2
  wires:
  Fx/1 -> estimateFrictionCoefficient/1(Fx)
  Fz/1 -> estimateFrictionCoefficient/2(Fz)
  SR/1 -> estimateFrictionCoefficient/3(SR)
  estimateFrictionCoefficient/1(mu) -> mu/1
  estimateFrictionCoefficient/2(normLongTireForce) -> normLongTireForce/1

== system TV2016/CarMaker/Estimations/selectVelocity ==
  v_est_x : Inport
  sensors : Inport  Port=2
  Bus Selector : BusSelector  OutputSignals=V_x_INS,V_x_optical
  Bus Selector1 : BusSelector  OutputSignals=V_y_INS,V_y_optical
  Constant1 : Constant  Value=settings.select_velocity_vx
  Constant2 : Constant  Value=settings.select_velocity_vy
  Index Vector : MultiPortSwitch
  Index Vector1 : MultiPortSwitch  DataPortOrder=Specify indices  Inputs=2  DataPortIndices={2,3}
  v_x : Outport
  v_y : Outport  Port=2
  wires:
  Constant1/1 -> Index Vector/1
  v_est_x/1 -> Index Vector/2
  sensors/1 -> Bus Selector1/1, Bus Selector/1
  Bus Selector/1 -> Index Vector/3  "<V_x_INS>"
  Bus Selector/2 -> Index Vector/4  "<V_x_optical>"
  Index Vector/1 -> v_x/1
  Constant2/1 -> Index Vector1/1
  Bus Selector1/1 -> Index Vector1/2  "<V_y_INS>"
  Bus Selector1/2 -> Index Vector1/3  "<V_y_optical>"
  Index Vector1/1 -> v_y/1

== system TV2016/CarMaker/IPG Vehicle/Brake ==
  note: <Your model here>
  note: When replacing the entire braking system,
      | be sure to add '-disablebrake' to the command line arguments
      | in the CarMaker Model Configuration block.
  Sync_In : Inport
  Brake.IF.In : Inport  Port=2
  VhclCtrl.Brake : Inport  Port=3
  Brake : S-Function  FunctionName=CM_Sfun  Parameters='Brake'
  BrakeUpd : S-Function  FunctionName=CM_Sfun  Parameters='BrakeUpd'
  BusCreator : BusCreator  Inputs=12
  CreateBus Vhcl.Wheel.PT : Subsystem
  Demux : Demux  Outputs=12
  Sync_Out : Outport
  Vhcl.Wheel.PT : Outport  Port=2
  wires:
  BrakeUpd/1 -> Sync_Out/1
  Brake/1 -> BrakeUpd/1  "Sync"
  Brake.IF.In/1 -> Brake/2
  VhclCtrl.Brake/1 -> Brake/3
  Brake/2 -> Demux/1
  BusCreator/1 -> BrakeUpd/2
  Sync_In/1 -> Brake/1
  Demux/12 -> BusCreator/12  "Brake IF Trq_Reg_trg RR"
  Demux/11 -> BusCreator/11  "Brake IF Trq_Reg_trg RL"
  Demux/10 -> BusCreator/10  "Brake IF Trq_Reg_trg FR"
  Demux/9 -> BusCreator/9  "Brake IF Trq_Reg_trg FL"
  Demux/8 -> BusCreator/8  "Brake IF Trq_PB RR"
  Demux/7 -> BusCreator/7  "Brake IF Trq_PB RL"
  Demux/6 -> BusCreator/6  "Brake IF Trq_PB FR"
  Demux/5 -> BusCreator/5  "Brake IF Trq_PB FL"
  Demux/4 -> BusCreator/4  "Brake IF Trq_WB RR"
  Demux/3 -> BusCreator/3  "Brake IF Trq_WB RL"
  Demux/2 -> BusCreator/2  "Brake IF Trq_WB FR"
  Demux/1 -> BusCreator/1  "Brake IF Trq_WB FL"
  BrakeUpd/2 -> CreateBus Vhcl.Wheel.PT/1(In)
  CreateBus Vhcl.Wheel.PT/1(Out) -> Vhcl.Wheel.PT/1

== system TV2016/CarMaker/IPG Vehicle/CarAndTrailer ==
  Sync_In : Inport
  VhclCtrl.Steering : Inport  Port=2
  Vhcl.Wheel.In : Inport  Port=3
  Vhcl.Misc : Inport  Port=4
  CarAndTrailerUpd : Subsystem
  Forces : Subsystem
  Ground : Ground
  Kinematics : Subsystem
  Kinetics : Subsystem
  Steering : Subsystem
  Terminator : Terminator
  Terminator1 : Terminator
  Trailer : Subsystem
  Sync_Out : Outport
  Brake.IF.In : Outport  Port=2
  wires:
  Trailer/9(Car.Hitch.FrcTrq) -> CarAndTrailerUpd/9(Car.Hitch.FrcTrq)
  Trailer/8(Vhcl.Wheel.RR) -> CarAndTrailerUpd/8(Vhcl.Wheel.RR)
  Trailer/7(Vhcl.Wheel.RL) -> CarAndTrailerUpd/7(Vhcl.Wheel.RL)
  Trailer/6(Vhcl.Wheel.FR) -> CarAndTrailerUpd/6(Vhcl.Wheel.FR)
  Trailer/5(Vhcl.Wheel.FL) -> CarAndTrailerUpd/5(Vhcl.Wheel.FL)
  Trailer/4(Vhcl.PoI) -> CarAndTrailerUpd/4(Vhcl.PoI)
  Trailer/3(Vhcl.Motion) -> CarAndTrailerUpd/3(Vhcl.Motion)
  Trailer/2(Vhcl.Steering) -> CarAndTrailerUpd/2(Vhcl.Steering)
  Trailer/1(Sync_Out) -> CarAndTrailerUpd/1(Sync_In)
  CarAndTrailerUpd/2(Brake.IF.In) -> Brake.IF.In/1
  CarAndTrailerUpd/1(Sync_Out) -> Sync_Out/1
  Vhcl.Misc/1 -> Terminator1/1
  Vhcl.Wheel.In/1 -> Terminator/1
  Kinetics/6(WheelCarrier.Misc) -> Trailer/6(WheelCarrier.Misc)
  Kinetics/5(Car.Trq_T2W) -> Trailer/5(Car.Trq_T2W)
  Steering/2(Steer.IF) -> Kinematics/2(Steer.IF)
  Kinetics/4(Car.Fr1) -> Trailer/4(Car.Fr1)
  Kinetics/3(Car.Hitch) -> Trailer/3(Car.Hitch)
  Kinetics/2(Trailer.Load) -> Trailer/2(Trailer.Load)
  VhclCtrl.Steering/1 -> Steering/2(VhclCtrl.Steering)
  Sync_In/1 -> Steering/1(Sync_In)
  Steering/1(Sync_Out) -> Kinematics/1(Sync_In)
  Kinetics/1(Sync_Out) -> Trailer/1(Sync_In)
  Ground/1 -> CarAndTrailerUpd/10(Vhcl.Fr1A)
  Forces/11(FStabi) -> Kinetics/11(FStabi)
  Forces/10(FDamp) -> Kinetics/10(FDamp)
  Forces/9(FSpring) -> Kinetics/9(FSpring)
  Forces/8(TireRR_Out) -> Kinetics/8(TireRR.Out)
  Forces/7(TireRL_Out) -> Kinetics/7(TireRL.Out)
  Forces/6(TireFR_Out) -> Kinetics/6(TireFR.Out)
  Forces/5(TireFL_Out) -> Kinetics/5(TireFL.Out)
  Forces/4(Car.Load) -> Kinetics/4(Car.Load)
  Forces/2(Car.Virtual) -> Kinetics/2(Car.Virtual)
  Kinematics/6(lSpring) -> Forces/6(lSpring)
  Kinematics/7(vDamp) -> Forces/7(vDamp)
  Forces/3(Car.Aero) -> Kinetics/3(Car.Aero)
  Forces/1(Sync_Out) -> Kinetics/1(Sync_In)
  Kinematics/5(TireRR_In) -> Forces/5(TireRR_In)
  Kinematics/4(TireRL_In) -> Forces/4(TireRL_In)
  Kinematics/3(TireFR_In) -> Forces/3(TireFR_In)
  Kinematics/2(TireFL_In) -> Forces/2(TireFL_In)
  Kinematics/1(Sync_Out) -> Forces/1(Sync_In)
  Kinematics/8(lStabi) -> Forces/8(lStabi)
  Forces/12(FBuf) -> Kinetics/12(FBuf)
  Kinematics/9(lBuf) -> Forces/9(lBuf)

== system TV2016/CarMaker/IPG Vehicle/PowerTrain ==
  note: When replacing the entire powertrain,
      | be sure to add '-disablepowertrain' to the command line arguments
      | in the CarMaker Model Configuration block.
  Sync_In : Inport
  Vhcl.Wheel.PT : Inport  Port=2
  VhclCtrl.PT : Inport  Port=3
  BusCreator : BusCreator  Inputs=40
  Demux : Demux  Outputs=40
  Electric Powertrain : Subsystem
  PowerTrain : S-Function  FunctionName=CM_Sfun  Parameters='PowerTrain'
  PowerTrainUpd : S-Function  FunctionName=CM_Sfun  Parameters='PowerTrainUpd'
  Terminator{1..6} (6 alike) : Terminator
  Sync_Out : Outport
  wires:
  Sync_In/1 -> PowerTrain/1
  PowerTrain/2 -> Demux/1
  PowerTrainUpd/1 -> Sync_Out/1
  PowerTrain/1 -> PowerTrainUpd/1  "Sync"
  Demux/1 -> BusCreator/1  "PT IF Ignition"
  Demux/2 -> Terminator2/1  "PT IF OperationState"
  Demux/4 -> ?  "PT IF GearNo"
  Demux/5 -> Terminator1/1  "PT IF Engine_rotv"
  Demux/7 -> ?  "PT IF Trq_Supp2Bdy1 x"
  Demux/8 -> ?  "PT IF Trq_Supp2Bdy1 y"
  Demux/9 -> ?  "PT IF Trq_Supp2Bdy1 z"
  Demux/10 -> ?  "PT IF Trq_Supp2BdyEng x"
  Demux/11 -> ?  "PT IF Trq_Supp2BdyEng y"
  Demux/12 -> ?  "PT IF DL_iDiff_mean"
  Demux/13 -> BusCreator/13  "PT IF WFL rot"
  Demux/14 -> BusCreator/14  "PT IF WFL rotv"
  Demux/15 -> ?  "PT IF WFL Trq_B2W"
  Demux/16 -> Terminator6/1  "PT IF WFL Trq_Drive"
  Demux/17 -> ?  "PT IF WFL Trq_Supp2WC"
  Demux/18 -> ?  "PT IF WFL Trq_BrakeReg"
  Demux/19 -> ?  "PT IF WFL Trq_BrakeReg_max"
  Demux/20 -> BusCreator/20  "PT IF WFR rot"
  Demux/21 -> BusCreator/21  "PT IF WFR rotv"
  Demux/22 -> ?  "PT IF WFR Trq_B2W"
  Demux/23 -> Terminator5/1  "PT IF WFR Trq_Drive"
  Demux/24 -> ?  "PT IF WFR Trq_Supp2WC"
  Demux/25 -> ?  "PT IF WFR Trq_BrakeReg"
  Demux/26 -> ?  "PT IF WFR Trq_BrakeReg_max"
  Demux/27 -> BusCreator/27  "PT IF WRL rot"
  Demux/28 -> BusCreator/28  "PT IF WRL rotv"
  Demux/29 -> ?  "PT IF WRL Trq_B2W"
  Demux/30 -> Terminator4/1  "PT IF WRL Trq_Drive"
  Demux/31 -> ?  "PT IF WRL Trq_Supp2WC"
  Demux/32 -> ?  "PT IF WRL Trq_BrakeReg"
  Demux/33 -> ?  "PT IF WRL Trq_BrakeReg_max"
  Demux/34 -> BusCreator/34  "PT IF WRR rot"
  Demux/35 -> BusCreator/35  "PT IF WRR rotv"
  Demux/36 -> ?  "PT IF WRR Trq_B2W"
  Demux/37 -> Terminator3/1  "PT IF WRR Trq_Drive"
  Demux/38 -> ?  "PT IF WRR Trq_Supp2WC"
  Demux/39 -> ?  "PT IF WRR Trq_BrakeReg"
  Demux/40 -> ?  "PT IF WRR Trq_BrakeReg_max"
  VhclCtrl.PT/1 -> PowerTrain/3
  Vhcl.Wheel.PT/1 -> PowerTrain/2
  BusCreator/1 -> PowerTrainUpd/2
  Electric Powertrain/2(PT.Engine.rotv) -> ?
  Demux/6 -> ?  "PT IF Engine_Trq (EngineControl)"
  Demux/3 -> BusCreator/3  "PT IF OperationError"
  Electric Powertrain/1(PT.OperationState) -> BusCreator/2
  Electric Powertrain/3(T_FL) -> BusCreator/16
  Electric Powertrain/4(T_FR) -> BusCreator/23
  Electric Powertrain/5(T_RL) -> BusCreator/30
  Electric Powertrain/6(T_RR) -> BusCreator/37

== system TV2016/CarMaker/Sensors /"Measured Power" ==
  RPM_FL : Inport
  RPM_FR : Inport  Port=2
  RPM_RL : Inport  Port=3
  RPM_RR : Inport  Port=4
  T_measured : Inport  Port=5
  2-D Lookup Table{,1..3} (4 alike) : Lookup_n-D  BreakpointsForDimension1=single([1.3,2.7,5.4,7.9,10.4,12.5,14.4,16.0,17.4,18.5,19.6]);  BreakpointsForDimension2=single([500,1000,2000,3000,4000,6000,10000,12000,15000,19000]);  Table=single(reshape([0.6437000036239624,0.5799999833106995,0.44999998807907104,0.3499999940395355,0.28999999165534973,0.23999999463558197,0.20000000298023224,0.17000000178813934,0.14000000059604645,0.12999999523162842,0.10999999940395355,0.7099999785423279,0.699999988079071,0.6100000143051148,0.5099999904632568,0.4399999976158142,0.3799999952316284,0.33000001311302185,0.28999999165534973,0.25,0.2199999988079071,0.20000000298023224,0.7300000190734863,0.7699999809265137,0.7300000190734863,0.6700000166893005,0.6100000143051148,0.550000011920929,0.5,0.44999998807907104,0.4000000059604645,0.36000001430511475,0.33000001311302185,0.7400000095367432,0.800000011920929,0.7900000214576721,0.7400000095367432,0.6899999976158142,0.6399999856948853,0.5899999737739563,0.5400000214576721,0.5,0.46000000834465027,0.41999998688697815,0.75,0.8199999928474426,0.8199999928474426,0.7799999713897705,0.7400000095367432,0.699999988079071,0.6600000262260437,0.6100000143051148,0.5699999928474426,0.5299999713897705,0.49000000953674316,0.7599999904632568,0.8399999737739563,0.8500000238418579,0.8299999833106995,0.800000011920929,0.7699999809265137,0.7400000095367432,0.699999988079071,0.6600000262260437,0.6200000047683716,0.5899999737739563,0.7699999809265137,0.8500000238418579,0.8799999952316284,0.8700000047683716,0.8600000143051148,0.8399999737739563,0.8100000023841858,0.7799999713897705,0.7599999904632568,0.7200000286102295,0.699999988079071,0.7699999809265137,0.8500000238418579,0.8899999856948853,0.8799999952316284,0.8700000047683716,0.8500000238418579,0.8299999833106995,0.8100000023841858,0.7799999713897705,0.7599999904632568,0.7300000190734863,0.7699999809265137,0.8600000143051148,0.8999999761581421,0.8999999761581421,0.8899999856948853,0.8700000047683716,0.8500000238418579,0.8299999833106995,0.8100000023841858,0.7900000214576721,0.6700000166893005,0.7799999713897705,0.8600000143051148,0.8999999761581421,0.9100000262260437,0.8999999761581421,0.8899999856948853,0.8700000047683716,0.8600000143051148,0.8299999833106995,0.7699999809265137,0.699999988079071],11,10));  ExtrapMethod=Clip  UseLastTableValue=on  InternalRulePriority=Speed  RndMeth=Simplest  InputSameDT=on
  Abs{,1..3} (4 alike) : Abs
  Add : Sum  Inputs=++++
  Bus Creator : BusCreator  Inputs=8  OutDataTypeStr=Bus: PowerDebug
      settings: InheritFromInputs=off
  Divide{,1..3} (4 alike) : Product  Inputs=*/
  MATLAB Function : MATLAB Function  TreatAsAtomicUnit=on
  Product{,1..3} (4 alike) : Product
  Switch{,1..3} (4 alike) : Switch  Criteria=u2 > Threshold
  "Measured Power " : Outport
  powerDebug : Outport  Port=2
  wires:
  MATLAB Function/2(T_FL) -> Abs/1
  MATLAB Function/3(RPM_FL) -> 2-D Lookup Table/2
  MATLAB Function/5(T_FR) -> Abs1/1
  MATLAB Function/8(T_RL) -> Abs2/1
  MATLAB Function/11(T_RR) -> Abs3/1
  MATLAB Function/12(RPM_RR) -> 2-D Lookup Table3/2
  Abs/1 -> 2-D Lookup Table/1
  Abs1/1 -> 2-D Lookup Table1/1
  Abs2/1 -> 2-D Lookup Table2/1
  Abs3/1 -> 2-D Lookup Table3/1
  2-D Lookup Table/1 -> Divide/2, Product/2
  MATLAB Function/1(Pm_FL) -> Product/1, Switch/2, Divide/1, Bus Creator/1
  Add/1 -> "Measured Power "/1
  2-D Lookup Table1/1 -> Divide1/2, Product1/2
  2-D Lookup Table2/1 -> Product2/2, Divide2/2
  2-D Lookup Table3/1 -> Product3/2, Divide3/2
  MATLAB Function/7(Pm_RL) -> Switch2/2, Product2/1, Divide2/1, Bus Creator/5
  MATLAB Function/10(Pm_RR) -> Bus Creator/7, Switch3/2, Product3/1, Divide3/1
  Bus Creator/1 -> powerDebug/1
  T_measured/1 -> MATLAB Function/5(T)
  MATLAB Function/6(RPM_FR) -> 2-D Lookup Table1/2
  MATLAB Function/9(RPM_RL) -> 2-D Lookup Table2/2
  RPM_FL/1 -> MATLAB Function/1(RPM_FL_IN)
  RPM_FR/1 -> MATLAB Function/2(RPM_FR_IN)
  RPM_RL/1 -> MATLAB Function/3(RPM_RL_IN)
  RPM_RR/1 -> MATLAB Function/4(RPM_RR_IN)
  Divide/1 -> Switch/1
  Product/1 -> Switch/3
  MATLAB Function/4(Pm_FR) -> Bus Creator/3, Product1/1, Switch1/2, Divide1/1
  Divide1/1 -> Switch1/1
  Product1/1 -> Switch1/3
  Divide2/1 -> Switch2/1
  Product2/1 -> Switch2/3
  Divide3/1 -> Switch3/1
  Product3/1 -> Switch3/3
  Switch1/1 -> Bus Creator/4, Add/2  "Pe_FR"
  Switch3/1 -> Add/4, Bus Creator/8  "Pe_RR"
  Switch2/1 -> Bus Creator/6, Add/3  "Pe_RL"
  Switch/1 -> Bus Creator/2, Add/1  "Pe_FL"

== system TV2016/CarMaker/VehicleControl/CreateBus Vhcl.Misc ==
  In1 : Inport
  Bus Creator5 : BusCreator  Inputs=11
  Demux5 : Demux  Outputs=11
  Out1 : Outport
  wires:
  Demux5/11 -> Bus Creator5/11  "Vhcl Wind_vel_0 z"
  Demux5/10 -> Bus Creator5/10  "Vhcl Wind_vel_0 y"
  Demux5/9 -> Bus Creator5/9  "Vhcl Wind_vel_0 x"
  Demux5/8 -> Bus Creator5/8  "Vhcl DL2BdyEng y"
  Demux5/7 -> Bus Creator5/7  "Vhcl DL2BdyEng x"
  Demux5/6 -> Bus Creator5/6  "Vhcl TrqDL2Bdy1B z"
  Demux5/5 -> Bus Creator5/5  "Vhcl TrqDL2Bdy1B y"
  Demux5/4 -> Bus Creator5/4  "Vhcl TrqDL2Bdy1B x"
  Demux5/3 -> Bus Creator5/3  "Vhcl Trq_DL2Bdy1 z"
  In1/1 -> Demux5/1
  Bus Creator5/1 -> Out1/1
  Demux5/2 -> Bus Creator5/2  "Vhcl Trq_DL2Bdy1 y"
  Demux5/1 -> Bus Creator5/1  "Vhcl Trq_DL2Bdy1 x"

== system TV2016/CarMaker/VehicleControl/CreateBus Vhcl.Wheel.In ==
  In1 : Inport
  Bus Creator1 : BusCreator  Inputs=12
  Demux1 : Demux  Outputs=12
  Out1 : Outport
  wires:
  Demux1/12 -> Bus Creator1/12  "Vhcl Wheel RR rotv"
  Demux1/11 -> Bus Creator1/11  "Vhcl Wheel RR Trq_DL2WC"
  Demux1/10 -> Bus Creator1/10  "Vhcl Wheel RR Trq_B2WC"
  Demux1/9 -> Bus Creator1/9  "Vhcl Wheel RL rotv"
  Demux1/8 -> Bus Creator1/8  "Vhcl Wheel RL Trq_DL2WC"
  Demux1/7 -> Bus Creator1/7  "Vhcl Wheel RL Trq_B2WC"
  Demux1/6 -> Bus Creator1/6  "Vhcl Wheel FR rotv"
  Demux1/5 -> Bus Creator1/5  "Vhcl Wheel FR Trq_DL2WC"
  Demux1/4 -> Bus Creator1/4  "Vhcl Wheel FR Trq_B2WC"
  Demux1/3 -> Bus Creator1/3  "Vhcl Wheel FL rotv"
  In1/1 -> Demux1/1
  Bus Creator1/1 -> Out1/1
  Demux1/2 -> Bus Creator1/2  "Vhcl Wheel FL Trq_DL2WC"
  Demux1/1 -> Bus Creator1/1  "Vhcl Wheel FL Trq_B2WC"

== system TV2016/CarMaker/VehicleControl/CreateBus VhclCtrl ==
  In : Inport
  Add KERS : MATLAB Function  TreatAsAtomicUnit=on
  BusCreator : BusCreator  Inputs=29
  Constant : Constant  Value=Use_Joystick
  Constant1 : Constant  Value=Use_Joystick
  Constant2 : Constant  Value=Use_Joystick
  Data Type Conversion : DataTypeConversion  OutDataTypeStr=double
  Demux : Demux  Outputs=29
  RacingwheelInterface : Subsystem
  Switch : Switch  Criteria=u2 > Threshold
  Switch1 : Switch  Criteria=u2 > Threshold
  Switch2 : Switch  Criteria=u2 > Threshold
  Write CM Dict1 : CarMaker4SL/Write CM Dict  xname=KERS_pos  xsync=off
  Out : Outport
  wires:
  In/1 -> Demux/1
  BusCreator/1 -> Out/1
  Demux/1 -> BusCreator/1  "VhclCtrl SST"
  Demux/2 -> BusCreator/2  "VhclCtrl Key"
  Demux/3 -> BusCreator/3  "VhclCtrl UserSignal0"
  Demux/4 -> BusCreator/4  "VhclCtrl UserSignal1"
  Demux/5 -> BusCreator/5  "VhclCtrl UserSignal2"
  Demux/6 -> BusCreator/6  "VhclCtrl UserSignal3"
  Demux/7 -> BusCreator/7  "VhclCtrl UserSignal4"
  Demux/8 -> BusCreator/8  "VhclCtrl GearNo"
  Demux/9 -> BusCreator/9  "VhclCtrl SelectorCtrl"
  Demux/10 -> Add KERS/1(brake_pedal)  "VhclCtrl Brake"
  Demux/11 -> BusCreator/11  "VhclCtrl BrakePark"
  Demux/12 -> BusCreator/12  "VhclCtrl Clutch"
  Demux/13 -> Switch1/1  "VhclCtrl Gas"
  Demux/14 -> Switch/1  "VhclCtrl Steering Ang"
  Demux/15 -> BusCreator/15  "VhclCtrl Steering AngVel"
  Demux/16 -> BusCreator/16  "VhclCtrl Steering AngAcc"
  Demux/17 -> BusCreator/17  "VhclCtrl Steering Trq"
  Demux/18 -> BusCreator/18  "VhclCtrl Lights LowBeam"
  Demux/19 -> BusCreator/19  "VhclCtrl Lights HighBeam"
  Demux/20 -> BusCreator/20  "VhclCtrl Lights Daytime"
  Demux/21 -> BusCreator/21  "VhclCtrl Lights ParkL"
  Demux/22 -> BusCreator/22  "VhclCtrl Lights ParkR"
  Demux/23 -> BusCreator/23  "VhclCtrl Lights IndL"
  Demux/24 -> BusCreator/24  "VhclCtrl Lights IndR"
  Demux/25 -> BusCreator/25  "VhclCtrl Lights FogFrontL"
  Demux/26 -> BusCreator/26  "VhclCtrl Lights FogFrontR"
  Demux/27 -> BusCreator/27  "VhclCtrl Lights FogRear"
  Demux/28 -> BusCreator/28  "VhclCtrl Lights Brake"
  Demux/29 -> BusCreator/29  "VhclCtrl Lights Reverse"
  RacingwheelInterface/1("Steering ") -> Switch/3
  RacingwheelInterface/2(throttleinoput) -> Switch1/3
  Constant/1 -> Switch/2
  Constant1/1 -> Switch1/2
  Constant2/1 -> Switch2/2
  RacingwheelInterface/3(brake input) -> Switch2/3
  Switch/1 -> BusCreator/14
  Switch1/1 -> BusCreator/13
  Switch2/1 -> BusCreator/10
  Add KERS/1(KERS_pos) -> Data Type Conversion/1
  Data Type Conversion/1 -> Write CM Dict1/1
  Add KERS/2(brake_pos) -> Switch2/1

== system TV2016/CarMaker/VehicleControl/CreateBus VhclCtrl.PT ==
  In1 : Inport
  BusCreator : BusCreator  Inputs=11
  Demux : Demux  Outputs=11
  Out1 : Outport
  wires:
  In1/1 -> Demux/1
  BusCreator/1 -> Out1/1
  Demux/1 -> BusCreator/1  "VhclCtrl SST"
  Demux/2 -> BusCreator/2  "VhclCtrl Key"
  Demux/3 -> BusCreator/3  "VhclCtrl UserSignal0"
  Demux/4 -> BusCreator/4  "VhclCtrl UserSignal1"
  Demux/5 -> BusCreator/5  "VhclCtrl UserSignal2"
  Demux/6 -> BusCreator/6  "VhclCtrl UserSignal3"
  Demux/7 -> BusCreator/7  "VhclCtrl UserSignal4"
  Demux/8 -> BusCreator/8  "VhclCtrl GearNo"
  Demux/9 -> BusCreator/9  "VhclCtrl SelectorCtrl"
  Demux/10 -> BusCreator/10  "VhclCtrl Clutch"
  Demux/11 -> BusCreator/11  "VhclCtrl Gas"

== system TV2016/CarMaker/VehicleControl/CreateBus VhclCtrl.Steering ==
  In1 : Inport
  Bus Creator : BusCreator  Inputs=5
  Demux : Demux  Outputs=5
  Out1 : Outport
  wires:
  In1/1 -> Demux/1
  Bus Creator/1 -> Out1/1
  Demux/1 -> Bus Creator/1  "VhclCtrl Steering Ang"
  Demux/5 -> Bus Creator/5  "VhclCtrl Steering ByTrq"
  Demux/3 -> Bus Creator/3  "VhclCtrl Steering AngAcc"
  Demux/2 -> Bus Creator/2  "VhclCtrl Steering AngVel"
  Demux/4 -> Bus Creator/4  "VhclCtrl Steering Trq"

== system TV2016/CarMaker/Control_System /Control /Power Limit Torque Reduction Controller  ==
  states : Inport
  Abs : Abs
  Add : Sum
  Discrete PI controller : simulink/Continuous/PID Controller  Controller=PI  TimeDomain=Discrete-time  SampleTime=-1  IntegratorMethod=Forward Euler  FilterMethod=Forward Euler  Form=Parallel  UseFilter=on  ControllerParametersSource=internal  P=powerLimitControl.Kp  I=powerLimitControl.Ki  D=0  N=100  InitialConditionSource=internal  InitialConditionForIntegrator=0  InitialConditionForFilter=0  ExternalReset=none  LimitOutput=on  UpperSaturationLimit=powerLimitControl.upper_sat_limit  LowerSaturationLimit=powerLimitControl.lower_sat_limit  LinearizeAsGain=off  AntiWindupMode=clamping  Kb=settings.Kb_EL;  TrackingMode=off  Kt=1  PParamMin=[]  PParamMax=[]  IParamMin=[]  IParamMax=[]  DParamMin=[]  DParamMax=[]  NParamMin=[]  NParamMax=[]  KbParamMin=[]  KbParamMax=[]  KtParamMin=[]  KtParamMax=[]  POutMin=[]  POutMax=[]  IOutMin=[]  IOutMax=[]  DOutMin=[]  DOutMax=[]  NOutMin=[]  NOutMax=[]  KbOutMin=[]  KbOutMax=[]  KtOutMin=[]  KtOutMax=[]  IntegratorOutMin=[]  IntegratorOutMax=[]  FilterOutMin=[]  FilterOutMax=[]  SumOutMin=[]  SumOutMax=[]  SumI1OutMin=[]  SumI1OutMax=[]  SumI2OutMin=[]  SumI2OutMax=[]  SumI3OutMin=[]  SumI3OutMax=[]  SumDOutMin=[]  SumDOutMax=[]  SaturationOutMin=[]  SaturationOutMax=[]  IntegratorContinuousStateAttributes=''  IntegratorStateMustResolveToSignalObject=off  IntegratorRTWStateStorageClass=Auto  FilterContinuousStateAttributes=''  FilterStateMustResolveToSignalObject=off  FilterRTWStateStorageClass=Auto  DifferentiatorICPrevScaledInput=0  DifferentiatorOutMin=[]  DifferentiatorOutMax=[]
  Index Vector : MultiPortSwitch  DataPortOrder=Zero-based contiguous  Inputs=2  zeroidx=on
  Negative Power limit : Constant  Value=powerLimitControl.negative_power_limit
  "Positive Power limit " : Constant  Value=powerLimitControl.positive_power_limit
  Red factor2 : Scope
      settings: ShowLegends=on  TimeRange=10  YMin=19.95  YMax=22.05  SaveName=ScopeData38
  Sum : Sum  Inputs=|+-
  Switch : Switch  Criteria=u2 > Threshold
  constant : Constant  Value=single(1)
  constant1 : Constant  Value=powerLimitControl.enable
  constant2 : Constant  Value=single(1)
  extractPower : MATLAB Function  TreatAsAtomicUnit=on
  Reduction Factor : Outport
  wires:
  extractPower/1(power) -> Red factor2/1, Abs/1, Switch/2
  Sum/1 -> Discrete PI controller/1
  Discrete PI controller/1 -> Add/2
  constant/1 -> Add/1
  Add/1 -> Index Vector/3
  states/1 -> extractPower/1(states)
  "Positive Power limit "/1 -> Switch/1
  Negative Power limit/1 -> Switch/3
  Switch/1 -> Sum/1
  Abs/1 -> Sum/2
  constant1/1 -> Index Vector/1
  constant2/1 -> Index Vector/2
  Index Vector/1 -> Reduction Factor/1
